simulink model "HeliRHONNControl"  (R2025a)
settings: Solver=FixedStepAuto  StartTime=0.0  StopTime=20  FixedStep=.001  MaxStep=1e-3  RelTol=1e-4  AbsTol=1e-6
values from neighbouring files (symbols this model uses):
  g = 9.81    [setup_heli_2d_configuration.m]
  J_eq_p = J_m_p + J_body_p + J_p + J_y    (= 0.0384309870395)    [setup_heli_2d_configuration.m]
  J_eq_y = J_m_y + J_body_y + J_p + J_y + J_shaft    (= 0.0431517259335)    [setup_heli_2d_configuration.m]
  K_pp = K_f_p * r_p    (= 0.20413345)    [setup_heli_2d_configuration.m]
  K_py = K_t_y / R_m_y    (= 0.0068125)    [setup_heli_2d_configuration.m]
  K_yp = K_t_p / R_m_p    (= 0.0219277108434)    [setup_heli_2d_configuration.m]
  K_yy = K_f_y * r_y    (= 0.071988045)    [setup_heli_2d_configuration.m]
  l_cm = ( (m_motor_p + m_shield ) * r_p +  (m_motor_y + m_shield ) * r_y ) / ( m_props )    (= 0.185670125995)    [setup_heli_2d_configuration.m]
  m_heli = 1.3872    [setup_heli_2d_configuration.m]
  p1 = 5.43784e+06    (= 5437840)    [Parametros.m]
  P1 = eye(2)*5e2    [Parametros.m]
  p2 = 83917.5    [Parametros.m]
  P2 = eye(2)*5e2    [Parametros.m]
  p3 = 1295.03    [Parametros.m]
  P3 = eye(2)*5e2    [Parametros.m]
  P4 = eye(2)*5e2    [Parametros.m]
  y1 = 75314.8    [Parametros.m]
  y2 = 9764.78    [Parametros.m]
  y3 = 1266.03    [Parametros.m]
undefined symbols (not defined in the file or in its folder): B_p, B_y, P12, P22, P32, P42, theta_0, VMAX_UPM_P, VMAX_UPM_Y, wk, wk2
libraries: simulink x2
settings Model: Creator=aceve  LastModifiedBy=aceve
settings DataIOCC: SaveFormat=StructureWithTime  SaveState=on

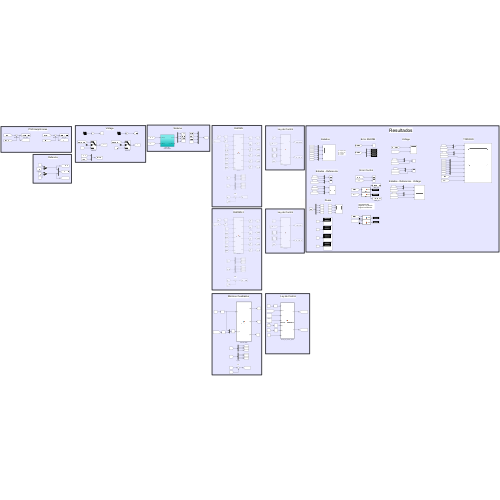
[thumbnail: Simulink's stored preview of the top-level diagram]
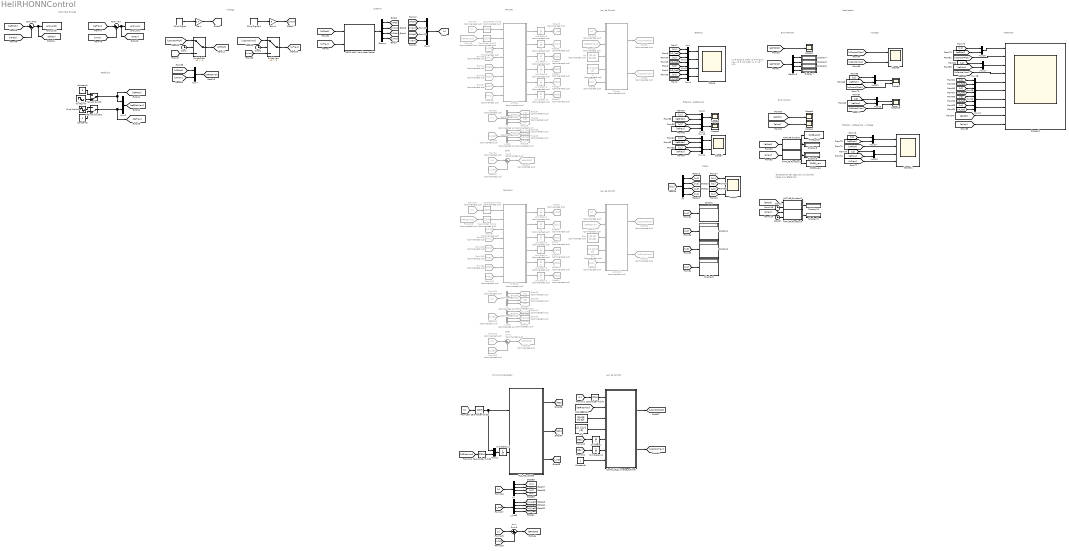
== system HeliRHONNControl ==
  note: Pesos
  note: Error RHONN
  note: Estados
  note: Voltage
  note: TODOOO
  note: Refencia
  note: PSO Help Errores
  note: Error Control
  note: Estados - Referencia
  note: error
  note: Resultados
  note: RHONN
  note: x1 = angulo pitch
      | x2 = angulo yaw
      | x3 = vel pitch
      | x4 = vel yaw
  note: Ley de Control
  note: Voltage
  note: Sistema
  note: Estados - Referencia - Voltage
  note: Ley de Control
  note: RHONN 2
  note: error
  note: error
  note: empezando del segundo 1.5 (donde llega a la referencia
  note: Minimos Cuadrados
  note: Ley de Control
  (0.45sin(t) : Sin  Amplitude=.45  SampleTime=0
  2DOF HELI: Nonlinear Model : Subsystem
  Chirp Signal : simulink/Sources/Chirp Signal  f1=.08  T=10  f2=1
  Chirp Signal1 : simulink/Sources/Chirp Signal  f1=.08  T=10  f2=1
  Clock{,1..3} (4 alike) : Clock
  Constant1 : Constant  Value=.8
  Constant2 : Constant  Value=4
  Constant5 : Constant
  Control : MATLAB Function  Commented=on  TreatAsAtomicUnit=on
  Control2 : MATLAB Function  Commented=on  TreatAsAtomicUnit=on
  Control_RLS_inverse_optimal : MATLAB Function  TreatAsAtomicUnit=on
  Demux : Demux
  Demux2 : Demux
  Display{,1..11} (12 alike) : Display
  Error Pitch : Sum  Inputs=|+-
  Error Yaw : Sum  Inputs=|+-
  From100 : From  Commented=on  GotoTag=P4k1
  From{8,19,39,42,45,101,104,107} (8 alike) : From  Commented=on  GotoTag=x
  From{35,40,43,97,102,105} (6 alike) : From  Commented=on  GotoTag=x_hat
  From103 : From  Commented=on  GotoTag=P1k1
  From106 : From  Commented=on  GotoTag=P2k1
  From108 : From  Commented=on  GotoTag=uFPitchYaw
  From22 : From  Commented=on  GotoTag=refPitchYaw
  From23 : From  Commented=on  GotoTag=refPitchYaw
  From{3,36,96,98} (4 alike) : From  Commented=on  GotoTag=wk1
  From37 : From  Commented=on  GotoTag=P3k1
  From38 : From  Commented=on  GotoTag=P4k1
  From41 : From  Commented=on  GotoTag=P1k1
  From44 : From  Commented=on  GotoTag=P2k1
  From46 : From  Commented=on  GotoTag=uFPitchYaw
  From99 : From  Commented=on  GotoTag=P3k1
  Gain : Gain  Gain=1.4
  Gain1 : Gain  Gain=5
  Goto23 : Goto  Commented=on  GotoTag=x_hat
  Goto24 : Goto  Commented=on  GotoTag=x2
  Goto25 : Goto  Commented=on  GotoTag=x4
  Goto26 : Goto  Commented=on  GotoTag=x3
  Goto27 : Goto  Commented=on  GotoTag=x2_hat
  Goto28 : Goto  Commented=on  GotoTag=x4_hat
  Goto29 : Goto  Commented=on  GotoTag=x3_hat
  Goto30 : Goto  Commented=on  GotoTag=x1_hat
  Goto31 : Goto  Commented=on  GotoTag=eRHONN
  Goto32 : Goto  Commented=on  GotoTag=wk1
  Goto33 : Goto  Commented=on  GotoTag=P1k1
  Goto34 : Goto  Commented=on  GotoTag=P2k1
  Goto35 : Goto  Commented=on  GotoTag=P3k1
  Goto36 : Goto  Commented=on  GotoTag=P4k1
  Goto37 : Goto  Commented=on  GotoTag=x1
  Goto38 : Goto  Commented=on  GotoTag=x2
  Goto39 : Goto  Commented=on  GotoTag=x4
  Goto40 : Goto  Commented=on  GotoTag=x3
  Goto41 : Goto  Commented=on  GotoTag=x2_hat
  Goto42 : Goto  Commented=on  GotoTag=x4_hat
  Goto43 : Goto  Commented=on  GotoTag=x3_hat
  Goto44 : Goto  Commented=on  GotoTag=x1_hat
  Goto45 : Goto  Commented=on  GotoTag=eRHONN
  Goto46 : Goto  Commented=on  GotoTag=wk1
  Goto47 : Goto  Commented=on  GotoTag=P1k1
  Goto48 : Goto  Commented=on  GotoTag=P2k1
  Goto49 : Goto  Commented=on  GotoTag=P3k1
  Goto5 : Goto  Commented=on  GotoTag=x_hat
  Goto50 : Goto  Commented=on  GotoTag=P4k1
  Goto51 : Goto  Commented=on  GotoTag=x1
  Goto52 : Goto  Commented=on  GotoTag=uControlYaw
  Goto53 : Goto  Commented=on  GotoTag=uControlPitch
  Goto8 : Goto  Commented=on  GotoTag=uControlYaw
  Goto9 : Goto  Commented=on  GotoTag=uControlPitch
  MATLAB Function : MATLAB Function  TreatAsAtomicUnit=on
  MATLAB Function1 : MATLAB Function  TreatAsAtomicUnit=on
  MATLAB Function2 : MATLAB Function  TreatAsAtomicUnit=on
  MATLAB Function3 : MATLAB Function  TreatAsAtomicUnit=on
  Manual Switch : ManualSwitch  CurrentSetting=0
  Manual Switch1 : ManualSwitch  CurrentSetting=0
  Mux{,1..4,7..22} (21 alike) : Mux  Inputs=2
  Mux6 : Mux
  Pp : Constant  Commented=on  Value=[p1 p2; p2 p3]
  Pp1 : Constant  Commented=on  Value=[p1 p2; p2 p3]
  Pp2 : Constant  Value=[p1 p2; p2 p3]
  Py : Constant  Commented=on  Value=[y1 y2;y2 y3]
  Py1 : Constant  Commented=on  Value=[y1 y2;y2 y3]
  Py2 : Constant  Value=[y1 y2;y2 y3]
  RHONN : MATLAB Function  Commented=on  TreatAsAtomicUnit=on
  RHONN2 : MATLAB Function  Commented=on  TreatAsAtomicUnit=on
  RLS_AB_update : MATLAB Function  TreatAsAtomicUnit=on
  RMSE_pitch : ToWorkspace  VariableName=RMSE_pitch  SaveFormat=Timeseries  SampleTime=-1
  RMSE_yaw : ToWorkspace  VariableName=RMSE_yaw  SaveFormat=Timeseries  SampleTime=-1
  Scope : Scope  NumInputPorts=4
      settings: ActiveDisplayString=4  Title=Vel Yaw  ActiveDisplayYMinimum=-0.7284950853697969  ActiveDisplayYMaximum=6.1765624842163289
  Scope{1,3..6} (5 alike) : Scope
      Scope1 settings: ActiveDisplayYMinimum=-1.0356608608631606  ActiveDisplayYMaximum=1.160288431182338
      Scope3 settings: ActiveDisplayYMinimum=-0.16814164905281398  ActiveDisplayYMaximum=1.5818583124773733  DataLoggingVariableName=ScopeData3
      Scope4 settings: ActiveDisplayYMinimum=0.38271741406841164  ActiveDisplayYMaximum=1.5375931509475163  DataLoggingVariableName=ScopeData4
      Scope5 settings: ActiveDisplayYMinimum=-1.0356608608631606  ActiveDisplayYMaximum=1.160288431182338  DataLoggingVariableName=ScopeData5
      Scope6 settings: ActiveDisplayYMinimum=-1.0356608608631606  ActiveDisplayYMaximum=1.160288431182338  DataLoggingVariableName=ScopeData6
  Scope{7..10} (4 alike) : Scope  NumInputPorts=2
      Scope10 settings: ActiveDisplayYMinimum=-1.0356608608631606  ActiveDisplayYMaximum=1.160288431182338  DataLoggingVariableName=ScopeData9
      Scope7 settings: Title=Pitch  ActiveDisplayYMinimum=-0.8514656404304296  ActiveDisplayYMaximum=0.594607293296831  DataLoggingVariableName=ScopeData7
      Scope8 settings: ActiveDisplayYMinimum=-0.00016635958558448762  ActiveDisplayYMaximum=0.00018560106830808887  DataLoggingVariableName=ScopeData8
      Scope9 settings: ActiveDisplayYMinimum=-1.0356608608631606  ActiveDisplayYMaximum=1.160288431182338  DataLoggingVariableName=ScopeData10
  Scope11 : Scope  NumInputPorts=4
      settings: ActiveDisplayYMinimum=-0.88357293382212931  ActiveDisplayYMaximum=0.88357293382212931  DataLoggingVariableName=ScopeData11
  Scope12 : Scope  NumInputPorts=10
      settings: ActiveDisplayYMinimum=-0.88271563659824781  ActiveDisplayYMaximum=0.87585725880719512  DataLoggingVariableName=ScopeData12
  Scope2 : Scope  NumInputPorts=4
      settings: ActiveDisplayYMinimum=-0.17717877234127791  ActiveDisplayYMaximum=1.3182422391794846  DataLoggingVariableName=ScopeData2
  Sine Wave1 : Sin  Amplitude=.9  Frequency=.5  Phase=pi/2  SampleTime=0
  Sum1 : Sum  Commented=on  Inputs=|+-
  Sum2 : Sum  Commented=on  Inputs=|+-
  Sum3 : Sum  Inputs=|+-
  SwitchPitch : Switch  Criteria=u2 > Threshold  Threshold=.1  SaturateOnIntegerOverflow=off  InputSameDT=off
  SwitchYaw : Switch  Criteria=u2 > Threshold  Threshold=.1  SaturateOnIntegerOverflow=off  InputSameDT=off
  Unit Delay : UnitDelay  SampleTime=-1  HasFrameUpgradeWarning=on
  Unit Delay1 : UnitDelay  Commented=on  InitialCondition=P42  SampleTime=-1  HasFrameUpgradeWarning=on
  Unit Delay10 : UnitDelay  Commented=on  InitialCondition=P4  SampleTime=-1  HasFrameUpgradeWarning=on
  Unit Delay11 : UnitDelay  SampleTime=-1  HasFrameUpgradeWarning=on
  Unit Delay12 : UnitDelay  SampleTime=-1  HasFrameUpgradeWarning=on
  Unit Delay2 : UnitDelay  Commented=on  SampleTime=-1  HasFrameUpgradeWarning=on
  Unit Delay3 : UnitDelay  Commented=on  InitialCondition=P12  SampleTime=-1  HasFrameUpgradeWarning=on
  Unit Delay4 : UnitDelay  Commented=on  InitialCondition=P22  SampleTime=-1  HasFrameUpgradeWarning=on
  Unit Delay5 : UnitDelay  Commented=on  InitialCondition=P32  SampleTime=-1  HasFrameUpgradeWarning=on
  Unit Delay6 : UnitDelay  Commented=on  SampleTime=-1  HasFrameUpgradeWarning=on
  Unit Delay7 : UnitDelay  Commented=on  InitialCondition=P1  SampleTime=-1  HasFrameUpgradeWarning=on
  Unit Delay8 : UnitDelay  Commented=on  InitialCondition=P2  SampleTime=-1  HasFrameUpgradeWarning=on
  Unit Delay9 : UnitDelay  Commented=on  InitialCondition=P3  SampleTime=-1  HasFrameUpgradeWarning=on
  Zero-Order Hold{1..4} (4 alike) : ZeroOrderHold  Commented=on  SampleTime=-1
  Zero-Order Hold5 : ZeroOrderHold  SampleTime=-1
  Zero-Order Hold6 : ZeroOrderHold  SampleTime=-1
  Zero-Order Hold7 : ZeroOrderHold  SampleTime=-1
  error_pitch : ToWorkspace  VariableName=error_pitch  SaveFormat=Timeseries  SampleTime=-1
  error_yaw : ToWorkspace  VariableName=error_yaw  SaveFormat=Timeseries  SampleTime=-1
  w1 : UnitDelay  Commented=on  InitialCondition=[wk]  SampleTime=-1  HasFrameUpgradeWarning=on
  w2 : UnitDelay  Commented=on  InitialCondition=[wk2]  SampleTime=-1  HasFrameUpgradeWarning=on
  wk : Demux
  x1 : Demux  Commented=on
  x2 : Demux  Commented=on
  x3 : Demux
  x_hat1 : Demux  Commented=on
  x_hat2 : Demux  Commented=on
  x_hat3 : Demux
  wires:
  [uControlPitch] -> Scope9/2
  x1/3 -> Goto26/1
  Unit Delay7/1 -> Goto33/1
  [uFYaw] -> 2DOF HELI: Nonlinear Model/2(u_yaw (V))
  x_hat1/4 -> Goto28/1
  [x1] -> Mux10/1
  From41/1 -> RHONN/5(P1k)
  Unit Delay6/1 -> Goto23/1
  [w2] -> Display1/1
  [xYaw] -> Error Yaw/2
  [x4_hat] -> Mux4/2
  Error Yaw/1 -> error_yaw/1, [eYaw]
  [x1] -> Mux16/1
  [refYaw] -> Mux9/2
  RHONN/3(P1k1) -> Unit Delay7/1
  Clock/1 -> SwitchPitch/2
  [x2] -> Mux19/1
  [x3_hat] -> Mux3/2
  Sum2/1 -> Goto31/1
  [eYaw] -> Scope4/1
  Pp/1 -> Control/3(Pp)
  Chirp Signal1/1 -> Gain1/1
  Mux7/1 -> [uFPitchYaw]
  [x2_hat] -> Mux1/2
  [x2] -> Mux9/1
  RHONN/4(P2k1) -> Unit Delay8/1
  Mux12/1 -> Scope9/1
  [xYaw] -> Mux6/2
  [x2] -> Mux1/1
  x_hat1/1 -> Goto30/1
  [wk1] -> wk/1
  [w3] -> Display2/1
  [x1] -> Mux/1
  Mux19/1 -> Scope12/6
  Mux15/1 -> Scope11/3
  Zero-Order Hold3/1 -> RHONN/2(u)
  Manual Switch1/1 -> [refYaw], Mux2/2
  [x2] -> Mux15/1
  RHONN/6(P4k1) -> Unit Delay10/1
  From23/1 -> Control/2(refPos)
  [eRHONN] -> Demux2/1
  [ePitch] -> Scope3/1
  Gain/1 -> [uPitch]
  Unit Delay9/1 -> Goto35/1
  From43/1 -> Sum2/2
  Mux/1 -> Scope/1
  Demux2/1 -> Display4/1
  [x1_hat] -> Mux/2
  [uFYaw] -> Mux7/2
  Py/1 -> Control/4(Py)
  [refPitch] -> Mux16/2
  Unit Delay10/1 -> Goto36/1
  [x3] -> Mux3/1
  Mux21/1 -> Scope12/8
  [refYaw] -> Mux17/2
  Demux2/2 -> Display5/1
  [x1] -> Mux12/1
  [x2] -> Mux13/1
  From44/1 -> RHONN/6(P2k)
  [x1] -> Mux8/1
  [uControlYaw] -> SwitchYaw/1
  [eYaw] -> Scope12/10
  Clock1/1 -> SwitchYaw/2
  wk/2 -> [w2]
  Demux2/4 -> Display7/1
  [refYaw] -> Mux11/2
  [refPitch] -> Mux10/2
  [ePitch] -> Scope12/9
  Mux1/1 -> Scope/2
  x1/2 -> Goto24/1
  From36/1 -> RHONN/4(wk)
  [refPitch] -> Mux14/2
  Sine Wave1/1 -> Manual Switch1/1
  RHONN/1(x_hat_k1) -> Unit Delay6/1
  [uFYaw] -> Scope11/4
  [uControlPitch] -> Scope12/2
  [uFPitch] -> Scope11/2
  From37/1 -> RHONN/7(P3k)
  From42/1 -> Sum2/1
  From3/1 -> Control/5(wk)
  Demux/4 -> [vYaw]
  Mux17/1 -> Scope12/3
  Mux14/1 -> Scope11/1
  [uControlPitch] -> SwitchPitch/1
  [x3] -> Mux20/1
  From45/1 -> Zero-Order Hold2/1
  [uControlYaw] -> Scope12/4
  [xPitch] -> Error Pitch/2
  Mux2/1 -> [refPitchYaw]
  From35/1 -> RHONN/3(x_hat)
  [uControlYaw] -> Scope8/2
  [uControlYaw] -> Scope10/2
  wk/4 -> [w4]
  RHONN/5(P3k1) -> Unit Delay9/1
  w1/1 -> Goto32/1
  [x3_hat] -> Mux20/2
  From39/1 -> x1/1
  [x2] -> Mux17/1
  Mux9/1 -> Scope6/1
  [w4] -> Display3/1
  SwitchPitch/1 -> [uFPitch]
  x1/4 -> Goto25/1
  Mux13/1 -> Scope10/1
  [uFPitch] -> 2DOF HELI: Nonlinear Model/1(u_pitch (V))
  x_hat1/2 -> Goto27/1
  [eRHONN] -> Scope1/1
  Mux10/1 -> Scope7/1
  [x1] -> Mux18/1
  Mux6/1 -> [x]
  [x4_hat] -> Mux21/2
  [w2] -> Scope2/2
  [uYaw] -> SwitchYaw/3
  Mux18/1 -> Scope12/5
  wk/1 -> [w1]
  Manual Switch/1 -> Mux2/1, [refPitch]
  [w1] -> Display/1
  From46/1 -> Zero-Order Hold3/1
  Mux8/1 -> Scope5/1
  From40/1 -> x_hat1/1
  Unit Delay8/1 -> Goto34/1
  Error Pitch/1 -> error_pitch/1, [ePitch]
  Mux20/1 -> Scope12/7
  wk/3 -> [w3]
  [refPitch] -> Mux12/2
  [refYaw] -> Mux15/2
  Mux16/1 -> Scope12/1
  Chirp Signal/1 -> Gain/1
  [uPitch] -> SwitchPitch/3
  (0.45sin(t)/1 -> Manual Switch/2
  x_hat1/3 -> Goto29/1
  [uFPitch] -> Mux7/1
  From38/1 -> RHONN/8(P4k)
  [vPitch] -> Mux6/3
  [x4] -> Mux4/1
  [refYaw] -> Error Yaw/1
  Gain1/1 -> [uYaw]
  [uControlPitch] -> Scope8/1
  [x2_hat] -> Mux19/2
  SwitchYaw/1 -> [uFYaw]
  Mux3/1 -> Scope/3
  [x4] -> Mux21/1
  [vYaw] -> Mux6/4
  [x1] -> Mux14/1
  [x2] -> Mux11/1
  x1/1 -> Goto37/1
  [refPitch] -> Mux8/2
  [refPitch] -> Error Pitch/1
  Constant1/1 -> Manual Switch/1
  Mux4/1 -> Scope/4
  Demux2/3 -> Display6/1
  RHONN/2(wk1) -> w1/1
  [w4] -> Scope2/4
  [w1] -> Scope2/1
  Constant2/1 -> Manual Switch1/2
  Mux11/1 -> Scope7/2
  Zero-Order Hold2/1 -> RHONN/1(x)
  From19/1 -> Control/1(x)
  [x1_hat] -> Mux18/2
  [refYaw] -> Mux13/2
  [w3] -> Scope2/3
  [xPitch] -> Mux6/1
  2DOF HELI: Nonlinear Model/1(X_sim) -> Demux/1
  Demux/1 -> [xPitch]
  Demux/2 -> [xYaw]
  Demux/3 -> [vPitch]
  Control/1(up) -> Goto9/1
  Control/2(uy) -> Goto8/1
  x_hat2/2 -> Goto41/1
  From101/1 -> x2/1
  Control2/2(uy) -> Goto52/1
  Control2/1(up) -> Goto53/1
  From105/1 -> Sum1/2
  Sum1/1 -> Goto45/1
  Zero-Order Hold1/1 -> RHONN2/1(x)
  From96/1 -> Control2/5(wk)
  Unit Delay3/1 -> Goto47/1
  From103/1 -> RHONN2/5(P1k)
  Py1/1 -> Control2/4(Py)
  RHONN2/2(wk1) -> w2/1
  x2/2 -> Goto38/1
  From97/1 -> RHONN2/3(x_hat)
  From99/1 -> RHONN2/7(P3k)
  From22/1 -> Control2/2(refPos)
  Pp1/1 -> Control2/3(Pp)
  x_hat2/3 -> Goto43/1
  x2/4 -> Goto39/1
  Zero-Order Hold4/1 -> RHONN2/2(u)
  x2/1 -> Goto51/1
  RHONN2/6(P4k1) -> Unit Delay1/1
  RHONN2/4(P2k1) -> Unit Delay4/1
  Unit Delay4/1 -> Goto48/1
  RHONN2/3(P1k1) -> Unit Delay3/1
  w2/1 -> Goto46/1
  From108/1 -> Zero-Order Hold4/1
  Unit Delay2/1 -> Goto5/1
  x_hat2/1 -> Goto44/1
  From102/1 -> x_hat2/1
  From106/1 -> RHONN2/6(P2k)
  From98/1 -> RHONN2/4(wk)
  x2/3 -> Goto40/1
  From8/1 -> Control2/1(x)
  RHONN2/5(P3k1) -> Unit Delay5/1
  From100/1 -> RHONN2/8(P4k)
  From104/1 -> Sum1/1
  Unit Delay5/1 -> Goto49/1
  x_hat2/4 -> Goto42/1
  Unit Delay1/1 -> Goto50/1
  From107/1 -> Zero-Order Hold1/1
  RHONN2/1(x_hat_k1) -> Unit Delay2/1
  [ePitch] -> MATLAB Function/1(e)
  [eYaw] -> MATLAB Function1/1(e)
  MATLAB Function1/1(RMSE) -> RMSE_yaw/1, Display9/1
  MATLAB Function/1(RMSE) -> RMSE_pitch/1, Display8/1
  Zero-Order Hold5/1 -> RLS_AB_update/1(x_k), Mux22/1
  [x] -> Zero-Order Hold5/1
  Zero-Order Hold7/1 -> Control_RLS_inverse_optimal/1(x)
  [x] -> Zero-Order Hold7/1
  [uFPitchYaw] -> Zero-Order Hold6/1
  [refPitchYaw] -> Control_RLS_inverse_optimal/2(refPos)
  x_hat3/3 -> [x3_hat]
  [x] -> Sum3/1
  x3/4 -> [x4]
  [x_hat] -> Sum3/2
  Sum3/1 -> [eRHONN]
  x_hat3/1 -> [x1_hat]
  x_hat3/4 -> [x4_hat]
  [x] -> x3/1
  x3/2 -> [x2]
  [x_hat] -> x_hat3/1
  x3/1 -> [x1]
  x3/3 -> [x3]
  x_hat3/2 -> [x2_hat]
  RLS_AB_update/1(ABp) -> [ABp]
  RLS_AB_update/2(ABy) -> [ABy]
  Pp2/1 -> Control_RLS_inverse_optimal/3(Pp)
  Py2/1 -> Control_RLS_inverse_optimal/4(Py)
  Constant5/1 -> Control_RLS_inverse_optimal/7(R)
  [ABp] -> Unit Delay/1
  Unit Delay/1 -> Control_RLS_inverse_optimal/5(ABp)
  [ABy] -> Unit Delay11/1
  Unit Delay11/1 -> Control_RLS_inverse_optimal/6(ABy)
  RLS_AB_update/3(x_hat) -> [x_hat]
  Unit Delay12/1 -> RLS_AB_update/2(x_u_ant)
  Mux22/1 -> Unit Delay12/1
  Zero-Order Hold6/1 -> Mux22/2
  MATLAB Function3/1(RMSE) -> Display11/1
  MATLAB Function2/1(RMSE) -> Display10/1
  [ePitch] -> MATLAB Function2/1(e)
  [eYaw] -> MATLAB Function3/1(e)
  Clock2/1 -> MATLAB Function2/2(t)
  Clock3/1 -> MATLAB Function3/2(t)
  Control_RLS_inverse_optimal/1(up) -> [uControlPitch]
  Control_RLS_inverse_optimal/2(uy) -> [uControlYaw]

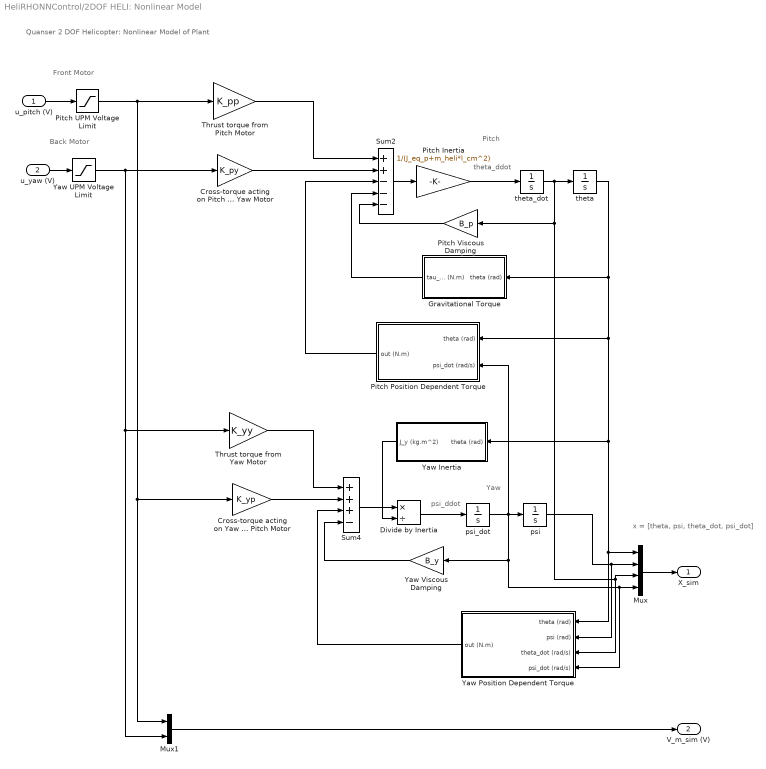
== system HeliRHONNControl/2DOF HELI: Nonlinear Model ==
  note: Back Motor
  note: Front Motor
  note: x = [theta, psi, theta_dot, psi_dot]
  note: Quanser 2 DOF Helicopter: Nonlinear Model of Plant
  note: theta_ddot
  note: psi_ddot
  note: Pitch
  note: Yaw
  u_pitch (V) : Inport
  u_yaw (V) : Inport  Port=2
  Cross-torque acting on Pitch from Yaw Motor : Gain  Gain=K_py
  Cross-torque acting on Yaw from Pitch Motor : Gain  Gain=K_yp
  Divide by Inertia : Product  Inputs=*/
  Gravitational Torque : Subsystem
  Mux : Mux
  Mux1 : Mux  Inputs=2
  Pitch Inertia : Gain  Gain=1/(J_eq_p+m_heli*l_cm^2)
  Pitch Position Dependent Torque : Subsystem  AncestorBlock=heli_2d_lib/2DOF Helicopter: Nonlinear Model/Yaw Nonlinear Element
  Pitch UPM Voltage Limit : Saturate  UpperLimit=VMAX_UPM_P  LowerLimit=- VMAX_UPM_P
  Pitch Viscous Damping : Gain  Gain=B_p
  Sum2 : Sum  Inputs=++---
  Sum4 : Sum  Inputs=+++-
  Thrust torque from Pitch Motor : Gain  Gain=K_pp
  Thrust torque from Yaw Motor : Gain  Gain=K_yy
  Yaw Inertia : Subsystem
  Yaw Position Dependent Torque : Subsystem
  Yaw UPM Voltage Limit : Saturate  UpperLimit=VMAX_UPM_Y  LowerLimit=- VMAX_UPM_Y
  Yaw Viscous Damping : Gain  Gain=B_y
  psi : Integrator
  psi_dot : Integrator
  theta : Integrator  InitialCondition=theta_0  LimitOutput=on  UpperSaturationLimit=40.5*pi/180  LowerSaturationLimit=-40.5*pi/180
  theta_dot : Integrator
  X_sim : Outport
  V_m_sim (V) : Outport  Port=2
  wires:
  Pitch Position Dependent Torque/1(out (N.m)) -> Sum2/3
  Gravitational Torque/1(tau_g (N.m)) -> Sum2/4
  Pitch Viscous Damping/1 -> Sum2/5
  Cross-torque acting on Pitch from Yaw Motor/1 -> Sum2/2
  Thrust torque from Pitch Motor/1 -> Sum2/1
  Yaw Inertia/1(J_y (kg.m^2)) -> Divide by Inertia/2
  Divide by Inertia/1 -> psi_dot/1
  Sum4/1 -> Divide by Inertia/1
  Yaw Position Dependent Torque/1(out (N.m)) -> Sum4/3
  Yaw Viscous Damping/1 -> Sum4/4
  psi/1 -> Yaw Position Dependent Torque/2(psi (rad)), Mux/2
  Mux1/1 -> V_m_sim (V)/1
  Yaw UPM Voltage Limit/1 -> Thrust torque from Yaw Motor/1, Mux1/2, Cross-torque acting on Pitch from Yaw Motor/1
  Pitch UPM Voltage Limit/1 -> Mux1/1, Cross-torque acting on Yaw from Pitch Motor/1, Thrust torque from Pitch Motor/1
  Mux/1 -> X_sim/1
  theta/1 -> Gravitational Torque/1(theta (rad)), Pitch Position Dependent Torque/1(theta (rad)), Yaw Position Dependent Torque/1(theta (rad)), Mux/1, Yaw Inertia/1(theta (rad))
  Sum2/1 -> Pitch Inertia/1
  Pitch Inertia/1 -> theta_dot/1
  theta_dot/1 -> Pitch Viscous Damping/1, Yaw Position Dependent Torque/3(theta_dot (rad/s)), Mux/3, theta/1
  Thrust torque from Yaw Motor/1 -> Sum4/1
  Cross-torque acting on Yaw from Pitch Motor/1 -> Sum4/2
  psi_dot/1 -> Yaw Viscous Damping/1, Yaw Position Dependent Torque/4(psi_dot (rad/s)), Mux/4, Pitch Position Dependent Torque/2(psi_dot (rad/s)), psi/1
  u_pitch (V)/1 -> Pitch UPM Voltage Limit/1
  u_yaw (V)/1 -> Yaw UPM Voltage Limit/1

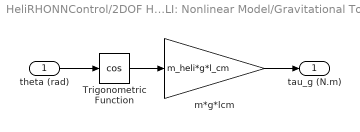
== system HeliRHONNControl/2DOF HELI: Nonlinear Model/Gravitational Torque ==
  theta (rad) : Inport
  Trigonometric Function : Trigonometry  Operator=cos  OutputSignalType=real
  m*g*lcm : Gain  Gain=m_heli*g*l_cm
  tau_g (N.m) : Outport
  wires:
  m*g*lcm/1 -> tau_g (N.m)/1
  theta (rad)/1 -> Trigonometric Function/1
  Trigonometric Function/1 -> m*g*lcm/1

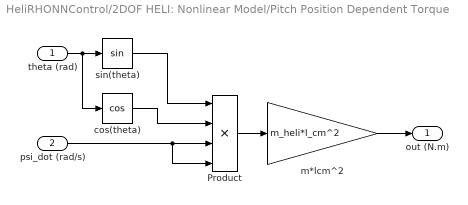
== system HeliRHONNControl/2DOF HELI: Nonlinear Model/Pitch Position Dependent Torque ==
  theta (rad) : Inport
  psi_dot (rad/s) : Inport  Port=2
  Product : Product  Inputs=4  RndMeth=Zero
  cos(theta) : Trigonometry  Operator=cos  OutputSignalType=real
  m*lcm^2 : Gain  Gain=m_heli*l_cm^2
  sin(theta) : Trigonometry  OutputSignalType=real
  out (N.m) : Outport
  wires:
  psi_dot (rad/s)/1 -> Product/4, Product/3
  theta (rad)/1 -> cos(theta)/1, sin(theta)/1
  Product/1 -> m*lcm^2/1
  sin(theta)/1 -> Product/1
  cos(theta)/1 -> Product/2
  m*lcm^2/1 -> out (N.m)/1

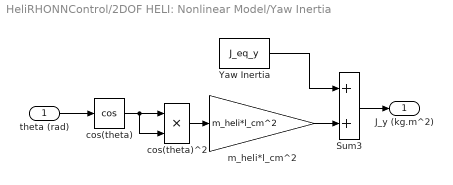
== system HeliRHONNControl/2DOF HELI: Nonlinear Model/Yaw Inertia ==
  theta (rad) : Inport
  Sum3 : Sum
  Yaw Inertia : Constant  Value=J_eq_y
  cos(theta) : Trigonometry  Operator=cos  OutputSignalType=real
  cos(theta)^2 : Product  RndMeth=Zero
  m_heli*l_cm^2 : Gain  Gain=m_heli*l_cm^2
  J_y (kg.m^2) : Outport
  wires:
  cos(theta)/1 -> cos(theta)^2/2, cos(theta)^2/1
  Sum3/1 -> J_y (kg.m^2)/1
  theta (rad)/1 -> cos(theta)/1
  m_heli*l_cm^2/1 -> Sum3/2
  Yaw Inertia/1 -> Sum3/1
  cos(theta)^2/1 -> m_heli*l_cm^2/1

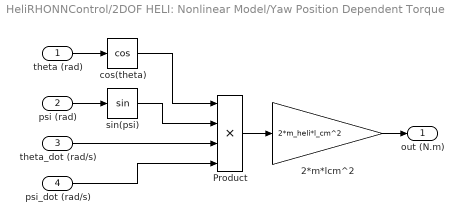
== system HeliRHONNControl/2DOF HELI: Nonlinear Model/Yaw Position Dependent Torque ==
  theta (rad) : Inport
  psi (rad) : Inport  Port=2
  theta_dot (rad/s) : Inport  Port=3
  psi_dot (rad/s) : Inport  Port=4
  2*m*lcm^2 : Gain  Gain=2*m_heli*l_cm^2
  Product : Product  Inputs=4  RndMeth=Zero
  cos(theta) : Trigonometry  Operator=cos  OutputSignalType=real
  sin(psi) : Trigonometry  OutputSignalType=real
  out (N.m) : Outport
  wires:
  2*m*lcm^2/1 -> out (N.m)/1
  psi_dot (rad/s)/1 -> Product/4
  theta_dot (rad/s)/1 -> Product/3
  sin(psi)/1 -> Product/2
  cos(theta)/1 -> Product/1
  Product/1 -> 2*m*lcm^2/1
  theta (rad)/1 -> cos(theta)/1
  psi (rad)/1 -> sin(psi)/1

== matlab function HeliRHONNControl/Control_RLS_inverse_optimal ==
  data: x input; up output; refPos input; Pp input; Py input; ABp input; ABy input; R input; uy output
function [up, uy] = Control_RLS_inverse_optimal(x, refPos, Pp, Py, ABp, ABy, R)
%#codegen
% Salidas escalares
up = 0.0; 
uy = 0.0;

% ---- Fuerza dimensiones y tipo ----
x      = reshape(double(x),     4,1);   % [theta_p; theta_y; omega_p; omega_y]
refPos = reshape(double(refPos),2,1);   % [r_pitch; r_yaw]
Pp     = reshape(double(Pp),     2,2);
Py     = reshape(double(Py),     2,2);
ABp    = reshape(double(ABp),    5,1);  % [a11 a12 a21 a22 bp]'
ABy    = reshape(double(ABy),    5,1);  % [a11 a12 a21 a22 by]'
R      = double(R);

% ---- Fuerza R escalar ----
if ~isscalar(R)
    R = R(1);        
end

% ---- Extrae modelos 2x2 por eje ----
A_p = [ABp(1) ABp(2);
       ABp(3) ABp(4)];
B_p = [0; ABp(5)];

A_y = [ABy(1) ABy(2);
       ABy(3) ABy(4)];
B_y = [0; ABy(5)];

% ---- Estados y referencias ----
xp = [x(1); x(3)];            % pitch: [pos; vel]
xy = [x(2); x(4)];            % yaw
rp = [refPos(1); 0];
ry = [refPos(2); 0];

% ---- f(x), g(x) lineales ----
fp = A_p*xp; gp = B_p;        % 2x1
fy = A_y*xy; gy = B_y;        % 2x1

% ---- Control inverso-óptimo (todo escalar) ----
epsR = 1e-12;

qpg   = 0.5*(gp.'*(Pp*gp));          % escalar
qyg   = 0.5*(gy.'*(Py*gy));          % escalar
num_p =        (gp.'*(Pp*(fp - rp)));% escalar
num_y =        (gy.'*(Py*(fy - ry)));% escalar

den_p = R + qpg;                     % escalar
den_y = R + qyg;                     % escalar

% Protecciones escalares
if (~isfinite(den_p)) || (den_p <= epsR)
    den_p = 1.0;
end
if (~isfinite(den_y)) || (den_y <= epsR)
    den_y = 1.0;
end

up = -0.5 * (num_p / den_p);         % escalar
uy = -0.5 * (num_y / den_y);         % escalar

end

== matlab function HeliRHONNControl/MATLAB Function2 ==
  settings: updateMethod=DISCRETE
  data: e input; RMSE output; t input
function RMSE = fcn(e, t)
% e: error escalar (por ejemplo, error_pitch o error_yaw)
% t: tiempo actual (s)
% RMSE: raíz del error cuadrático medio acumulada (escalar)

persistent S_E2 N
if isempty(S_E2)
    S_E2 = 0;
    N    = uint32(0);
end

if t >= 1.5  % empieza a contar desde 1.5 s
    e    = double(e);
    S_E2 = S_E2 + e.^2;
    N    = N + 1;
end

if N > 0
    RMSE = sqrt(S_E2 / double(N));
else
    RMSE = 0;
end
end

== matlab function HeliRHONNControl/MATLAB Function3 ==
  settings: updateMethod=DISCRETE
  data: e input; RMSE output; t input
function RMSE = fcn(e, t)
% e: error escalar (por ejemplo, error_pitch o error_yaw)
% t: tiempo actual (s)
% RMSE: raíz del error cuadrático medio acumulada (escalar)

persistent S_E2 N
if isempty(S_E2)
    S_E2 = 0;
    N    = uint32(0);
end

if t >= 1.5  % empieza a contar desde 1.5 s
    e    = double(e);
    S_E2 = S_E2 + e.^2;
    N    = N + 1;
end

if N > 0
    RMSE = sqrt(S_E2 / double(N));
else
    RMSE = 0;
end
end

== matlab function HeliRHONNControl/Control2 ==
  data: x input; refPos input; Pp input; Py input; wk input; up output; uy output
function [up, uy] = Control2(x, refPos, Pp, Py, wk)
% CONTROL2 – Ley de control para RHONN2 (16 pesos, 4 por estado).
% x      = [x1; x2; x3; x4]
% refPos = [r_pitch; r_yaw] (solo posición)
% Pp,Py  = matrices SPD 2x2 (pitch/yaw)
% wk     = [w1..w4 | w5..w8 | w9..w12 | w13..w16]' (16x1)
% O1,O2  = ganancias de entrada (por defecto 0.01 en RHONN2)
%
% Salida: up (para u1/pitch), uy (para u2/yaw)
O1 = 0.01;
O2 = 0.01;

    R = 1;                          % penalización escalar (puedes ajustar)
    epsR = 1e-9;                    % para robustez numérica

    % ===== mismas saturaciones suaves que RHONN2 =====
    xc = max(min(x,5),-5);
    x1 = xc(1); x2 = xc(2); x3 = xc(3); x4 = xc(4);

    % ===== partición de pesos (idéntica a RHONN2) =====
    w1 = wk(1:4);    % estado 1 (x1)
    w2 = wk(5:8);    % estado 2 (x2)
    w3 = wk(9:12);   % estado 3 (x3)
    w4 = wk(13:16);  % estado 4 (x4)

    % ===== dinámicas sin entrada (f) – exactamente como en RHONN2 =====
    % x_hat_1 (sin u)
    f1 = w1(1)*tanh(x3) ...
       + w1(2)*tanh(0.9*x1) ...
       + w1(3)*((x3 - x1)./(1+abs(x3 - x1))) ...
       + w1(4)*exp(-0.5*(x2/1.0)^2);

    % x_hat_2 (sin u)
    f2 = w2(1)*tanh(x4) ...
       + w2(2)*tanh(0.9*x2) ...
       + w2(3)*((x4 - x2)./(1+abs(x4 - x2))) ...
       + w2(4)*exp(-0.5*(x1/1.0)^2);

    % x_hat_3 (sin u)  (en RHONN2 lleva + O1*u1, aquí excluimos la entrada)
    f3 = w3(1)*tanh(0.8*x3) ...
       + w3(2)*tanh(0.6*x1) ...
       + w3(3)*log1p(exp(x3 - x1)) ...
       + w3(4)*exp(-0.5*(x4/1.0)^2);

    % x_hat_4 (sin u)  (en RHONN2 lleva + O2*u2, aquí excluimos la entrada)
    f4 = w4(1)*tanh(0.8*x4) ...
       + w4(2)*tanh(0.6*x2) ...
       + w4(3)*log1p(exp(x4 - x2)) ...
       + w4(4)*exp(-0.5*(x3/1.0)^2);

    % ===== agrupación por sub-sistema =====
    % Pitch: [x1; x3]  con entrada u1 => g_p = [0; O1]
    % Yaw:   [x2; x4]  con entrada u2 => g_y = [0; O2]
    fp = [f1; f3];
    gp = [0; O1];

    fy = [f2; f4];
    gy = [0; O2];

    % ===== referencias (posición + velocidad_ref=0) =====
    rp = [refPos(1); 0];
    ry = [refPos(2); 0];

    % ===== control óptimo instantáneo tipo cuadrático =====
    % u = -0.5 * (R + 0.5*g'Pg)^(-1) * (g'P(f - r))
    % (misma forma que usabas; se asegura simetría/robustez)
    Pp = (Pp + Pp.')/2;
    Py = (Py + Py.')/2;

    S_p = (R + 0.5*(gp.'*Pp*gp)) + epsR;
    S_y = (R + 0.5*(gy.'*Py*gy)) + epsR;

    up = -0.5 * ( (gp.'*Pp*(fp - rp)) / S_p );
    uy = -0.5 * ( (gy.'*Py*(fy - ry)) / S_y );
end

== matlab function HeliRHONNControl/RHONN ==
  data: x input; u input; x_hat_k1 output; x_hat input; wk input; P1k input; P2k input; wk1 output; P1k1 output; P2k1 output; P3k input; P4k input; P3k1 output; P4k1 output
function [x_hat_k1, wk1, P1k1, P2k1, P3k1, P4k1] = RHONN(x,u,x_hat,wk,P1k,P2k,P3k,P4k)
% Identificador RHONN con 4 EKF (uno por estado)
% x = [x1; x2; x3; x4], u = [u1; u2]
% wk = [w1 w2 | w3 w4 | w5 w6 | w7 w8]'

x_hat_k1 = zeros(4,1); wk1 = zeros(8,1);
P1k1 = zeros(2); P2k1 = zeros(2); P3k1 = zeros(2); P4k1 = zeros(2);


%% Ganancias constantes de entrada (ajustables)
O1 = 0.01;
O2 = 0.01;

%% Modelo neuronal (predicción x_hat(k+1))
x_hat_1 = wk(1)*tanh(x(3)) + wk(2)*tanh(x(1));
x_hat_2 = wk(3)*tanh(x(4)) + wk(4)*tanh(x(2));
x_hat_3 = wk(5)*tanh(x(3)) + wk(6)*tanh(x(1)) + O1*u(1);
x_hat_4 = wk(7)*tanh(x(4)) + wk(8)*tanh(x(2)) + O2*u(2);
x_hat_k1 = [x_hat_1; x_hat_2; x_hat_3; x_hat_4];

%% Regresores (derivadas parciales respecto a wk)
H1 = [tanh(x(3)) tanh(x(1))];
H2 = [tanh(x(4)) tanh(x(2))];
H3 = [tanh(x(3)) tanh(x(1))];
H4 = [tanh(x(4)) tanh(x(2))];

%% Covarianzas EKF
Q1 = eye(2)*5e2;  R1 = 6e3;
Q2 = eye(2)*1e2;  R2 = 6e1;
Q3 = eye(2)*5e2;  R3 = 6e3;
Q4 = eye(2)*5e2;  R4 = 6e2;

%% Innovación
e = x - x_hat;

%% EKF #1 (actualiza [w1 w2])
K1   = P1k*H1'/(R1 + H1*P1k*H1');
w1k1 = [wk(1); wk(2)] + K1*e(1);
P1k1 = P1k - K1*H1*P1k + Q1;

%% EKF #2 (actualiza [w3 w4])
K2   = P2k*H2'/(R2 + H2*P2k*H2');
w2k1 = [wk(3); wk(4)] + K2*e(2);
P2k1 = P2k - K2*H2*P2k + Q2;

%% EKF #3 (actualiza [w5 w6])
K3   = P3k*H3'/(R3 + H3*P3k*H3');
w3k1 = [wk(5); wk(6)] + K3*e(3);
P3k1 = P3k - K3*H3*P3k + Q3;

%% EKF #4 (actualiza [w7 w8])
K4   = P4k*H4'/(R4 + H4*P4k*H4');
w4k1 = [wk(7); wk(8)] + K4*e(4);
P4k1 = P4k - K4*H4*P4k + Q4;

%% Ensamble de pesos
wk1 = [w1k1; w2k1; w3k1; w4k1];



end

== matlab function HeliRHONNControl/Control ==
  data: x input; refPos input; Pp input; Py input; wk input; up output; uy output
function [up,uy] = Control(x,refPos,Pp,Py,wk)
% refPos = [r_pitch; r_yaw]  (solo posiciones)

% Model RHONN
w_1 = 0.01;  
w_2 = 0.01;

fp = [wk(1)*tanh(x(3)) + wk(2)*tanh(x(1));
      wk(5)*tanh(x(3)) + wk(6)*tanh(x(1))];
gp = [0; w_1];

fy = [wk(3)*tanh(x(4)) + wk(4)*tanh(x(2));
      wk(7)*tanh(x(4)) + wk(8)*tanh(x(2))];
gy = [0; w_2];

% Referencias solo de posición
rp = [refPos(1); 0];
ry = [refPos(2); 0];

% Ley de control
R  = 1;
up = -0.5*(R + 0.5*gp'*Pp*gp)\(gp'*Pp*(fp - rp));
uy = -0.5*(R + 0.5*gy'*Py*gy)\(gy'*Py*(fy - ry));
end

== matlab function HeliRHONNControl/RHONN2 ==
  data: x input; u input; x_hat_k1 output; x_hat input; wk input; P1k input; P2k input; wk1 output; P1k1 output; P2k1 output; P3k input; P4k input; P3k1 output; P4k1 output
function [x_hat_k1, wk1, P1k1, P2k1, P3k1, P4k1] = RHONN2(x,u,x_hat,wk,P1k,P2k,P3k,P4k)
% RHONN + 4 EKF (uno por estado) con 4 pesos/estado = 16 pesos total
% x=[x1;x2;x3;x4], u=[u1;u2], wk=[w1..w4|w5..w8|w9..w12|w13..w16]'

    % ===== Preasigna salidas con tamaño EXPLÍCITO =====
    x_hat_k1 = zeros(4,1, 'like', x);
    wk1      = zeros(16,1,'like', x);
    P1k1     = zeros(4,4, 'like', P1k);
    P2k1     = zeros(4,4, 'like', P2k);
    P3k1     = zeros(4,4, 'like', P3k);
    P4k1     = zeros(4,4, 'like', P4k);

    % ===== Ganancias de entrada (mismo tipo que x) =====
    O1 = cast(0.01, 'like', x);
    O2 = cast(0.01, 'like', x);




% === Ganancias de entrada (fijas) ===
O1 = 0.01; O2 = 0.01;

% (opcional) anti-saturación suave para las bases
xc = max(min(x,5),-5);



% === Bases (regresores) 1×4 por estado ===
H1 = [tanh(xc(3)), tanh(xc(1)), ((xc(3)-xc(1))./(1+abs(xc(3)-xc(1)))), exp(-0.5*(xc(2)/1.0)^2)];
H2 = [tanh(xc(4)), tanh(xc(2)), ((xc(4)-xc(2))./(1+abs(xc(4)-xc(2)))), exp(-0.5*(xc(1)/1.0)^2)];
H3 = [tanh(xc(3)), tanh(xc(1)), log1p(exp(xc(3)-xc(1))),              exp(-0.5*(xc(4)/1.0)^2)];
H4 = [tanh(xc(4)), tanh(xc(2)), log1p(exp(xc(4)-xc(2))),              exp(-0.5*(xc(3)/1.0)^2)];

% === Partición de pesos (4 por estado) ===
w1 = wk(1:4);   w2 = wk(5:8);   w3 = wk(9:12);   w4 = wk(13:16);

% === Predicción x_hat(k+1) con pesos "a priori" ===
x_hat_1 = w1(1)*tanh(xc(3)) + w1(2)*tanh(0.9*xc(1)) + w1(3)*((xc(3)-xc(1))./(1+abs(xc(3)-xc(1)))) + w1(4)*exp(-0.5*(xc(2)/1.0)^2);
x_hat_2 = w2(1)*tanh(xc(4)) + w2(2)*tanh(0.9*xc(2)) + w2(3)*((xc(4)-xc(2))./(1+abs(xc(4)-xc(2)))) + w2(4)*exp(-0.5*(xc(1)/1.0)^2);
x_hat_3 = w3(1)*tanh(0.8*xc(3)) + w3(2)*tanh(0.6*xc(1)) + w3(3)*log1p(exp(xc(3)-xc(1))) + w3(4)*exp(-0.5*(xc(4)/1.0)^2) + O1*u(1);
x_hat_4 = w4(1)*tanh(0.8*xc(4)) + w4(2)*tanh(0.6*xc(2)) + w4(3)*log1p(exp(xc(4)-xc(2))) + w4(4)*exp(-0.5*(xc(3)/1.0)^2) + O2*u(2);
x_hat_k1 = [x_hat_1; x_hat_2; x_hat_3; x_hat_4];

% === Innovación ===
e = x - x_hat;   % 4x1

% === Ruido proceso/medición (ajustables) ===
Q1 = eye(4)*1e2;  R1 = 1e3;
Q2 = eye(4)*1e2;  R2 = 1e3;
Q3 = eye(4)*1e2;  R3 = 1e3;
Q4 = eye(4)*1e2;  R4 = 1e3;

% === EKF por estado (H:1x4, P:4x4, K:4x1) ===
% #1
S1  = R1 + H1*P1k*H1.';
K1  = (P1k*H1.')/S1;
w1k1 = w1 + K1*e(1);
P1k1 = P1k - K1*(H1*P1k) + Q1;     % forma simple (puedes usar Joseph si quieres)

% #2
S2  = R2 + H2*P2k*H2.';
K2  = (P2k*H2.')/S2;
w2k1 = w2 + K2*e(2);
P2k1 = P2k - K2*(H2*P2k) + Q2;

% #3
S3  = R3 + H3*P3k*H3.';
K3  = (P3k*H3.')/S3;
w3k1 = w3 + K3*e(3);
P3k1 = P3k - K3*(H3*P3k) + Q3;

% #4
S4  = R4 + H4*P4k*H4.';
K4  = (P4k*H4.')/S4;
w4k1 = w4 + K4*e(4);
P4k1 = P4k - K4*(H4*P4k) + Q4;

% === Ensamble de pesos actualizados ===
wk1 = [w1k1; w2k1; w3k1; w4k1];
end

== matlab function HeliRHONNControl/MATLAB Function ==
  settings: updateMethod=DISCRETE
  data: e input; RMSE output
function RMSE = fcn(e)
% e: error escalar (por ejemplo, error_pitch o error_yaw)
% RMSE: raíz del error cuadrático medio acumulada (escalar)

persistent S_E2 N
if isempty(S_E2)
    S_E2 = 0;
    N    = uint32(0);
end

e    = double(e);   % asegura tipo
S_E2 = S_E2 + e.^2; % acumula e^2
N    = N + 1;       % cuenta muestras

RMSE = sqrt( S_E2 / max(1,double(N)) );
end

== matlab function HeliRHONNControl/MATLAB Function1 ==
  settings: updateMethod=DISCRETE
  data: e input; RMSE output
function RMSE = fcn(e)
% e: error escalar (por ejemplo, error_pitch o error_yaw)
% RMSE: raíz del error cuadrático medio acumulada (escalar)

persistent S_E2 N
if isempty(S_E2)
    S_E2 = 0;
    N    = uint32(0);
end

e    = double(e);   % asegura tipo
S_E2 = S_E2 + e.^2; % acumula e^2
N    = N + 1;       % cuenta muestras

RMSE = sqrt( S_E2 / max(1,double(N)) );
end

== matlab function HeliRHONNControl/RLS_AB_update ==
  data: x_k input; x_u_ant input; ABp output; ABy output; x_hat output
function [ABp, ABy, x_hat] = RLS_AB_update(x_k, x_u_ant)
%#codegen
% RLS Estructurado y Desacoplado para 2-DOF Heli
% x_k = [x1; x2; x3; x4] (Estado actual k, usado como TARGET 'y')
% x_u_ant = [x1_ant; x2_ant; x3_ant; x4_ant; u1_ant; u2_ant] (Datos en k-1, usado como REGRESOR 'phi')

%% --- Pre-inicialización de Salidas ---
ABp   = zeros(5, 1, 'double');
ABy   = zeros(5, 1, 'double');
x_hat = zeros(4, 1, 'double');

%% --- Parámetros RLS ---
lambda = 0.995;
P0     = 1e4;

% === Tamaños de Regresores ===
n_p1 = 2; % [x1_ant, x3_ant]
n_p2 = 3; % [x1_ant, x3_ant, u1_ant]
n_y1 = 2; % [x2_ant, x4_ant]
n_y2 = 3; % [x2_ant, x4_ant, u2_ant]

% === Variables Persistentes ===
persistent P_p1 P_p2 P_y1 P_y2 th_p1 th_p2 th_y1 th_y2
if isempty(P_p1)
    % Persistent para Pitch
    P_p1  = eye(n_p1) * P0;
    th_p1 = zeros(n_p1, 1);
    P_p2  = eye(n_p2) * P0;
    th_p2 = zeros(n_p2, 1);
    % Persistent para Yaw
    P_y1  = eye(n_y1) * P0;
    th_y1 = zeros(n_y1, 1);
    P_y2  = eye(n_y2) * P0;
    th_y2 = zeros(n_y2, 1);
end

%% --- Definición de Targets (y) y Regresores (phi) ---
% Extraer datos retrasados (k-1) del vector de entrada
x1_ant = x_u_ant(1);
x2_ant = x_u_ant(2);
x3_ant = x_u_ant(3);
x4_ant = x_u_ant(4);
u1_ant = x_u_ant(5);
u2_ant = x_u_ant(6);

% Targets 'y' (estado actual k)
y_p1 = x_k(1); % x1(k)
y_p2 = x_k(3); % x3(k)
y_y1 = x_k(2); % x2(k)
y_y2 = x_k(4); % x4(k)

% Regresores 'phi' (estado/control en k-1)
phi_p1 = [x1_ant; x3_ant];            % (n_p1 x 1)
phi_p2 = [x1_ant; x3_ant; u1_ant];    % (n_p2 x 1)
phi_y1 = [x2_ant; x4_ant];            % (n_y1 x 1)
phi_y2 = [x2_ant; x4_ant; u2_ant];    % (n_y2 x 1)

%% --- Actualización RLS (4 bloques) ---

% === RLS #1: Pitch Pos (x1) ===
den = lambda + (phi_p1.' * (P_p1 * phi_p1));
K   = (P_p1 * phi_p1) / den;
e   = y_p1 - phi_p1.' * th_p1;
th_p1 = th_p1 + K * e;
P_p1  = (P_p1 - K * (phi_p1.' * P_p1)) / lambda;

% === RLS #2: Pitch Vel (x3) ===
den = lambda + (phi_p2.' * (P_p2 * phi_p2));
K   = (P_p2 * phi_p2) / den;
e   = y_p2 - phi_p2.' * th_p2;
th_p2 = th_p2 + K * e;
P_p2  = (P_p2 - K * (phi_p2.' * P_p2)) / lambda;

% === RLS #3: Yaw Pos (x2) ===
den = lambda + (phi_y1.' * (P_y1 * phi_y1));
K   = (P_y1 * phi_y1) / den;
e   = y_y1 - phi_y1.' * th_y1;
th_y1 = th_y1 + K * e;
P_y1  = (P_y1 - K * (phi_y1.' * P_y1)) / lambda;

% === RLS #4: Yaw Vel (x4) ===
den = lambda + (phi_y2.' * (P_y2 * phi_y2));
K   = (P_y2 * phi_y2) / den;
e   = y_y2 - phi_y2.' * th_y2;
th_y2 = th_y2 + K * e;
P_y2  = (P_y2 - K * (phi_y2.' * P_y2)) / lambda;

%% --- Asignación de Salidas ---
% Parámetros para el controlador
% th_p1 = [a11_p; a12_p]
% th_p2 = [a21_p; a22_p; bp]
ABp(:) = [th_p1(1); th_p1(2); th_p2(1); th_p2(2); th_p2(3)];

% th_y1 = [a11_y; a12_y]
% th_y2 = [a21_y; a22_y; by]
ABy(:) = [th_y1(1); th_y1(2); th_y2(1); th_y2(2); th_y2(3)];

% Predicción (esta es la predicción de x(k) basada en los datos de k-1)
x_hat(:) = [phi_p1.' * th_p1;
            phi_y1.' * th_y1;
            phi_p2.' * th_p2;
            phi_y2.' * th_y2];
end
